simulink library "bcm"  (R2021b)
settings: Solver=VariableStepAuto  StartTime=0.0  StopTime=10.0  RelTol=1e-3
undefined symbols (not defined in the file or in its folder): ENUM_ANTITHEFT_ALARM, ENUM_ANTITHEFT_ARM, ENUM_ANTITHEFT_DISARM, ENUM_ANTITHEFT_WAIT, ENUM_GEARPOSNTOCAN_P, ENUM_PDKEYRAWLULOCK_INUNLOCK, ENUM_PDKEYRAWPS_INPS, ENUM_POWERSTA_ON, ENUM_POWERSTA_READY, ENUM_POWERSTA_STANDBY, ENUM_PWRSTASW_ON, ENUM_PWRSTASW_READY, ENUM_VEHICLETYPE_D21, ENUM_VEHICLETYPE_D31F25, ENUM_VEHICLETYPE_D31HAWD, ENUM_VEHICLETYPE_D31HRWD, ENUM_VEHICLETYPE_D31L24, FALSE, KBCM_ACCSwcPrsTmr_s, KBCM_ALMBrightnessDark_enum, KBCM_AmbBlue_enum, KBCM_AmbBreathT_ms, KBCM_AmbGreen_enum, KBCM_AmbMidPple_enum, KBCM_AmbRed_enum, KBCM_AmbTempCtrlEN_flg, KBCM_AmbTempT_s, KBCM_AmbWelModeENWait_s, KBCM_Antitheft_enum_ovrdflg, KBCM_Antitheft_enum_ovrdval, KBCM_APMDoorCtrlSta_flg_ovrdflg, KBCM_APMDoorCtrlSta_flg_ovrdval, KBCM_CmdKeepT_s, KBCM_CSWLightRstDebT_s, KBCM_CSWTurnLPRstT_s, KBCM_DelayTSW_flg, KBCM_DiagDRLOFF_flg, KBCM_DiagFLTC_mA, KBCM_DiagFMHT_s, KBCM_DiagFRTC_mA, KBCM_DiagRLTC_mA, KBCM_DiagRRTC_mA, KBCM_DrAPMRetryTimes_cnt, KBCM_DrOpenWdwOT_s, KBCM_DrOpenWdwReady_s, KBCM_ESSOffT_ms, KBCM_ESSOnT_ms, KBCM_FDCDKCReDetectT_K, KBCM_FDCDKCUSSFilterT_K, KBCM_HandleLampKeepT_s, KBCM_IVIRstHoldT_ms, KBCM_IVIRstTriggerT_ms, KBCM_ONDelayT_ms, KBCM_RAPSAbnFlashOFFT_ms, KBCM_RAPSAbnFlashONT_ms, KBCM_ReDetectT_K, KBCM_RightHandDriveEN_flg, KBCM_RLSLowSpdFilterT_s, KBCM_RmLampKeep_min, KBCM_RmLpKeyInT_s ... (+37)
libraries: simulink x389, $bdroot x11, hcu_lib x2
(part 4 of 13)

== system bcm/BCM/BCM/CenterDoorLock ==
  task_time_s : Inport
  VBCM_LockSetting_flg : Inport  Port=2
  VBCM_AntitheftSta_enum : Inport  Port=3
  VBCM_AllDoorSW_flg : Inport  Port=4  OutDataTypeStr=boolean
  VTQD_DiagHCrash_flg : Inport  Port=5
  VPMM_PwrSta_enum : Inport  Port=6
  VINP_CentralDoorLockSW_flg : Inport  Port=7
  VBCM_BCMDoorLockSta_flg : Inport  Port=8
  VBCM_ATActCtrl_enum : Inport  Port=9
  VINP_AirBagFailCmd_flg : Inport  Port=10
  VINP_VehSpeed_kph : Inport  Port=11
  VINP_funAuto_flg : Inport  Port=12
  VINP_CDLUnlockButt_flg : Inport  Port=13  OutDataTypeStr=boolean
  VINP_CDLLockButt_flg : Inport  Port=14  OutDataTypeStr=boolean
  VTQD_CrashDetd_flg : Inport  Port=15
  EEP_FuelDoorPos : Inport  Port=16
  VINP_FlashfUnlockSingle_flg : Inport  Port=17
  VINP_DrDoorSW_flg : Inport  Port=18
  VINP_PsDoorSW_flg : Inport  Port=19
  VINP_RLDoorSW_flg : Inport  Port=20
  VINP_RRDoorSW_flg : Inport  Port=21
  VINP_FLHandleClose_flg : Inport  Port=22
  VINP_FRHandleClose_flg : Inport  Port=23
  VINP_RLHandleClose_flg : Inport  Port=24
  VINP_RRHandleClose_flg : Inport  Port=25
  KBCM_CmdKeepT_s : Inport  Port=26
  KBCM_HandleLampKeepT_s : Inport  Port=27
  VTQD_ShiftGearPosn_enum : Inport  Port=28
  VBCM_AutoLockSta_flg : Inport  Port=29
  VBCM_AutoUnlockSta_flg : Inport  Port=30
  Chart : Stateflow chart  TreatAsAtomicUnit=on
      settings: PortSchema="{\"entries\":[{\"content\":{\"sides\":[{\"content\":{\"connectorIds\":[\"In24\",\"In1\",\"In2\",\"In3\",\"In25\",\"In29\",\"In26\",\"In27\",\"In28\",\"In4\",\"In5\",\"In6\",\"In7\",\"In8\",\"In9\",\"In10\",\"In11\",\"In12\",\"In13\",\"In16\",\"In19\",\"In20\",\"In22\",\"In17\",\"In18\",\"In21\",\"In23\",\"In14\",\"In15\"]},\"type\":\"ConnectorPlacement.EquallySpacedRectSide\",\"uuid\":\"d1cad239-ac39-46ec-a1da-ab943ad28110\"},{\"content\":{\"connectorIds\":[\"Out1\",\"Out2\",\"Out3\",\"Out4\",\"Out5\",\"Out6\",\"Out7\",\"Out8\",\"Out9\",\"Out10\"],\"side\":\"RIGHT\"},\"type\":\"ConnectorPlacement.EquallySpacedRectSide\",\"uuid\":\"4472ac08-1c38-4faf-8087-989b09b8fb8a\"},{\"content\":{\"connectorIds\":[],\"side\":\"TOP\"},\"type\":\"ConnectorPlacement.EquallySpacedRectSide\",\"uuid\":\"615ae9d4-02db-4768-8556-b21c6d1e705f\"}]},\"type\":\"ConnectorPlacement.EquallySpacedConnector\",\"uuid\":\"559c67f6-8021-453c-91d3-74fce83e0396\"}],\"packageUris\":[\"http://schema.mathworks.com/mf0/Connector/R2020b\"],\"version\":\"1.0\"}"
  Data Type Conversion : DataTypeConversion  OutDataTypeStr=boolean
  Data Type Conversion1 : DataTypeConversion  OutDataTypeStr=boolean
  Divide : Product  Inputs=*/
  Divide1 : Product  Inputs=*/
  Terminator : Terminator
  Unit Delay : UnitDelay  SampleTime=-1  HasFrameUpgradeWarning=on
  Unit Delay1 : UnitDelay  SampleTime=-1  HasFrameUpgradeWarning=on
  VBCM_FrChargingDoorCtrl_enum : Outport
  VBCM_RrChargingDoorCtrl_enum : Outport  Port=2
  VBCM_CrashDetd_flg : Outport  Port=3
  VBCM_CTDCtrl_enum : Outport  Port=4
  DoorLockIND : Outport  Port=5
  VBCM_fVIGHandle_flg : Outport  Port=6
  VBCM_CTDLockSW_flg : Outport  Port=7
  VBCM_FuelDoorPos_flg : Outport  Port=8
  VBCM_DiagHCrash_flg : Outport  Port=9
  VBCM_fUnlockSingle_flg : Outport  Port=10
  VBCM_FDLHandleLampCmd_flg : Outport  Port=11
  VBCM_FDRHandleLampCmd_flg : Outport  Port=12
  VBCM_FDHandleCmd_enum : Outport  Port=13
  wires:
  VBCM_AntitheftSta_enum/1 -> Chart/1(AntitheftSta)
  VINP_CDLUnlockButt_flg/1 -> Chart/9(CDL_Unlock_Butt)
  Chart/5(fVIGHandle) -> VBCM_fVIGHandle_flg/1  "VBCM_fVIGHandle_flg"
  VINP_funAuto_flg/1 -> Terminator/1
  VINP_VehSpeed_kph/1 -> Chart/8(VehSpeed)
  VINP_AirBagFailCmd_flg/1 -> Chart/7(AirBagFailCmd)
  VBCM_ATActCtrl_enum/1 -> Chart/6(ATLockCtrl)
  Chart/4(DoorLockIND) -> DoorLockIND/1  "VBCM_DoorLockIND_flg"
  VBCM_AllDoorSW_flg/1 -> Chart/2(AllDoorSW)
  Chart/1(FrChargingDoorCtrl) -> VBCM_FrChargingDoorCtrl_enum/1  "VBCM_FrChargingDoorCtrl_enum"
  Chart/2(RrChargingDoorCtrl) -> VBCM_RrChargingDoorCtrl_enum/1  "VBCM_RrChargingDoorCtrl_enum"
  VBCM_BCMDoorLockSta_flg/1 -> Chart/5(BCM_DoorLock_Sta)
  VBCM_LockSetting_flg/1 -> Chart/24(LockSetting)  "VINP_SetUnlockSingle_flg"
  Chart/3(CTDCtrl) -> VBCM_CTDCtrl_enum/1  "VBCM_CTDCtrl_enum"
  VINP_CDLLockButt_flg/1 -> Chart/10(CDL_Lock_Butt)
  [CTDLockSW] -> VBCM_CTDLockSW_flg/1  "VBCM_CTDLockSW_flg"
  VPMM_PwrSta_enum/1 -> [VPMM_PwrSta_enum]  "VPMM_PwrSta_enum"
  [VPMM_PwrSta_enum] -> Chart/3(PwrSta), Unit Delay/1
  VTQD_CrashDetd_flg/1 -> [VBCM_CrashDetd_flg]
  VINP_CentralDoorLockSW_flg/1 -> [CTDLockSW]  "VINP_CentralDoorLockSwSG09_flg"
  [CTDLockSW] -> Chart/4(CentralDoorLockSW)
  Data Type Conversion/1 -> VBCM_DiagHCrash_flg/1  "VBCM_DiagHCrash_flg"
  Data Type Conversion1/1 -> VBCM_CrashDetd_flg/1  "VBCM_CrashDetd_flg"
  VTQD_DiagHCrash_flg/1 -> Data Type Conversion/1
  [VBCM_CrashDetd_flg] -> Data Type Conversion1/1
  EEP_FuelDoorPos/1 -> Chart/12(EEP_FuelDoorPos)
  Chart/6(FuelDoorPos) -> VBCM_FuelDoorPos_flg/1  "VBCM_FuelDoorPos_flg"
  Chart/7(fUnlockSingle) -> VBCM_fUnlockSingle_flg/1  "VBCM_fUnlockSingle_flg"
  VINP_FlashfUnlockSingle_flg/1 -> Chart/13(VINP_FlashfUnlockSingle_flg)
  Chart/8(VBCM_FDLHandleLampCmd_flg) -> VBCM_FDLHandleLampCmd_flg/1
  Chart/9(VBCM_FDRHandleLampCmd_flg) -> VBCM_FDRHandleLampCmd_flg/1
  VINP_DrDoorSW_flg/1 -> Chart/16(VINP_DrDoorSW_flg)
  VINP_PsDoorSW_flg/1 -> Chart/19(VINP_PsDoorSW_flg)
  VINP_RLDoorSW_flg/1 -> Chart/20(VINP_RLDoorSW_flg)
  VINP_RRDoorSW_flg/1 -> Chart/22(VINP_RRDoorSW_flg)
  VINP_FLHandleClose_flg/1 -> Chart/17(VINP_FLHandleClose_flg)
  VINP_FRHandleClose_flg/1 -> Chart/18(VINP_FRHandleClose_flg)
  VINP_RLHandleClose_flg/1 -> Chart/21(VINP_RLHandleClose_flg)
  VINP_RRHandleClose_flg/1 -> Chart/23(VINP_RRHandleClose_flg)
  [task_time_s] -> Divide/2
  KBCM_HandleLampKeepT_s/1 -> Divide1/1
  [task_time_s] -> Divide1/2
  KBCM_CmdKeepT_s/1 -> Divide/1
  Divide/1 -> Chart/14(KBCM_CmdKeepT_s)
  Divide1/1 -> Chart/15(KBCM_HandleLampKeepT_s)
  Chart/10(VBCM_FDHandleCmd_enum) -> VBCM_FDHandleCmd_enum/1
  task_time_s/1 -> [task_time_s]
  Unit Delay/1 -> Chart/25(PwrStaBuf)
  VTQD_ShiftGearPosn_enum/1 -> Unit Delay1/1, Chart/29(VTQD_ShiftGearPosn_enum)
  Unit Delay1/1 -> Chart/26(ShiftGearPosnBuf)
  VBCM_AutoUnlockSta_flg/1 -> Chart/28(VBCM_AutoUnlockSta_flg)
  VBCM_AutoLockSta_flg/1 -> Chart/27(VBCM_AutoLockSta_flg)
  [VBCM_CrashDetd_flg] -> Chart/11(CrashDetd)

== system bcm/BCM/BCM/DID Judgement ==
  VINP_DiagFMHT_s : Inport
  VINP_DiagFLTC_mA : Inport  Port=2
  VINP_DiagFRTC_mA : Inport  Port=3
  VINP_DiagRLTC_mA : Inport  Port=4
  VINP_DiagRRTC_mA : Inport  Port=5
  VINP_DiagDRLOFF_flg : Inport  Port=6
  VINP_VehicleType_enum : Inport  Port=7
  Add1 : Sum
  Constant{,6,8,10,12,14} (6 alike) : Constant  Value=ENUM_VEHICLETYPE_D31L24
  Constant1 : Constant  Value=ENUM_VEHICLETYPE_D31HRWD
  Constant16 : Constant  Value=ENUM_VEHICLETYPE_D31F25
  Constant18 : Constant  Value=KBCM_DiagDRLOFF_flg
  Constant4 : Constant  Value=KBCM_TurnLPErrEN_flg
  Constant44 : Constant  Value=KBCM_DiagFMHT_s
  Constant45 : Constant  Value=10
  Constant46 : Constant  Value=KBCM_DiagFLTC_mA
  Constant47 : Constant  Value=KBCM_DiagFRTC_mA
  Constant48 : Constant  Value=KBCM_DiagRLTC_mA
  Constant49 : Constant  Value=KBCM_DiagRRTC_mA
  Constant7 : Constant  Value=ENUM_VEHICLETYPE_D31HAWD
  Equal{,2..9} (9 alike) : RelationalOperator  Operator===  OutDataTypeStr=boolean  RndMeth=Simplest
  Gain{,2..4} (4 alike) : Gain  Gain=10
  Gain1 : Gain  Gain=5
  Logical Operator : Logic  Operator=OR  Inputs=4  AllPortsSameDT=off  OutDataTypeStr=boolean
  Switch{,2..6} (6 alike) : Switch  Criteria=u2 > Threshold
  VBCM_DiagFMHT_s : Outport
  VBCM_DiagFLTC_mA : Outport  Port=2
  VBCM_DiagFRTC_mA : Outport  Port=3
  VBCM_DiagRLTC_mA : Outport  Port=4
  VBCM_DiagRRTC_mA : Outport  Port=5
  VBCM_DiagDRLOFF_flg : Outport  Port=6
  VBCM_TurnLPErrEN_flg : Outport  Port=7
  wires:
  Constant47/1 -> Gain2/1
  Gain1/1 -> Add1/1
  Constant45/1 -> Add1/2
  Constant49/1 -> Gain4/1
  Constant44/1 -> Gain1/1
  Constant48/1 -> Gain3/1
  Constant46/1 -> Gain/1
  [VINP_DiagFMHT_s] -> Switch/1
  Equal/1 -> Switch/2
  Add1/1 -> Switch/3
  Switch/1 -> VBCM_DiagFMHT_s/1  "VBCM_DiagFMHT_s"
  Switch6/1 -> VBCM_DiagFLTC_mA/1  "VBCM_DiagFLTC_mA"
  [VINP_DiagFLTC_mA] -> Switch6/1
  Switch2/1 -> VBCM_DiagFRTC_mA/1  "VBCM_DiagFRTC_mA"
  Gain2/1 -> Switch2/3
  [VINP_DiagFRTC_mA] -> Switch2/1
  Gain3/1 -> Switch3/3
  [VINP_DiagRLTC_mA] -> Switch3/1
  Switch3/1 -> VBCM_DiagRLTC_mA/1  "VBCM_DiagRLTC_mA"
  Gain4/1 -> Switch4/3
  [VINP_DiagRRTC_mA] -> Switch4/1
  Switch4/1 -> VBCM_DiagRRTC_mA/1  "VBCM_DiagRRTC_mA"
  Logical Operator/1 -> Switch5/2
  [VINP_DiagDRLOFF_flg] -> Switch5/1
  Switch5/1 -> VBCM_DiagDRLOFF_flg/1  "VBCM_DiagDRLOFF_flg"
  Constant18/1 -> Switch5/3
  VINP_DiagFMHT_s/1 -> [VINP_DiagFMHT_s]
  VINP_DiagFLTC_mA/1 -> [VINP_DiagFLTC_mA]
  VINP_DiagFRTC_mA/1 -> [VINP_DiagFRTC_mA]
  VINP_DiagRLTC_mA/1 -> [VINP_DiagRLTC_mA]
  VINP_DiagRRTC_mA/1 -> [VINP_DiagRRTC_mA]
  VINP_DiagDRLOFF_flg/1 -> [VINP_DiagDRLOFF_flg]
  Constant/1 -> Equal/2
  Constant6/1 -> Equal7/2
  Equal2/1 -> Switch2/2
  Constant8/1 -> Equal2/2
  Equal4/1 -> Switch3/2
  Constant12/1 -> Equal4/2
  Equal3/1 -> Switch4/2
  Constant10/1 -> Equal3/2
  Equal5/1 -> Logical Operator/1
  Constant14/1 -> Equal5/2
  Equal6/1 -> Logical Operator/2
  Constant16/1 -> Equal6/2
  VINP_VehicleType_enum/1 -> [VINP_VehicleType_enum]
  [VINP_VehicleType_enum] -> Equal/1
  [VINP_VehicleType_enum] -> Equal2/1
  [VINP_VehicleType_enum] -> Equal4/1
  [VINP_VehicleType_enum] -> Equal3/1
  [VINP_VehicleType_enum] -> Equal5/1
  [VINP_VehicleType_enum] -> Equal6/1
  [VINP_VehicleType_enum] -> Equal8/1
  Constant1/1 -> Equal8/2
  Constant7/1 -> Equal9/2
  [VINP_VehicleType_enum] -> Equal9/1
  Equal9/1 -> Logical Operator/4
  Equal8/1 -> Logical Operator/3
  Equal7/1 -> Switch6/2
  [VINP_VehicleType_enum] -> Equal7/1
  Gain/1 -> Switch6/3
  Constant4/1 -> VBCM_TurnLPErrEN_flg/1

== system bcm/BCM/BCM/Dimmer ==
  VINP_MFRDNBrightReq_pct : Inport
  VINP_IVIStatus_flg : Inport  Port=2
  VINP_IVINightModeSta_flg : Inport  Port=3
  VBCM_PosLamp_flag : Inport  Port=4
  VINP_CANMsgValidIVI2_flg : Inport  Port=5
  EEP_MFRDNBrightReq : Inport  Port=6
  BCMInitial : Inport  Port=7
  Chart : Stateflow chart  TreatAsAtomicUnit=on
      settings: PortSchema="{\"entries\":[{\"content\":{\"sides\":[{\"content\":{\"connectorIds\":[\"In4\",\"In1\",\"In2\",\"In3\"]},\"type\":\"ConnectorPlacement.EquallySpacedRectSide\",\"uuid\":\"076f305a-8f7e-4e65-8c9e-aa6699a69b21\"},{\"content\":{\"connectorIds\":[\"Out1\",\"Out2\"],\"side\":\"RIGHT\"},\"type\":\"ConnectorPlacement.EquallySpacedRectSide\",\"uuid\":\"bf947e95-3d60-4849-99c4-9fb941c8d282\"},{\"content\":{\"side\":\"TOP\"},\"type\":\"ConnectorPlacement.EquallySpacedRectSide\",\"uuid\":\"13c4efb7-da15-49ea-8253-a9d27aa3456c\"}]},\"type\":\"ConnectorPlacement.EquallySpacedConnector\",\"uuid\":\"7282b60f-551e-46a0-a3a5-beda89adbd0d\"}],\"packageUris\":[\"http://schema.mathworks.com/mf0/Connector/R2020b\"],\"version\":\"1.0\"}"
  Data Type Conversion1 : DataTypeConversion
  Switch1 : Switch  Criteria=u2 > Threshold
  Switch2 : Switch  Criteria=u2 > Threshold
  Switch3 : Switch  Criteria=u2 > Threshold
  Unit Delay : UnitDelay  SampleTime=-1  HasFrameUpgradeWarning=on
  Unit Delay1 : UnitDelay  SampleTime=-1  HasFrameUpgradeWarning=on
  VBCM_Dimmer_pct : Outport
  VBCM_DimmerEN_flg : Outport  Port=2
  VBCM_MFRDNBrightReq_pct : Outport  Port=3
  wires:
  VBCM_PosLamp_flag/1 -> Chart/3(PLamp)
  Chart/1(Dimmer) -> VBCM_Dimmer_pct/1  "VBCM_Dimmer_pct"
  VINP_IVIStatus_flg/1 -> Chart/1(IVI_Status)
  Chart/2(DimmerEN) -> VBCM_DimmerEN_flg/1  "VBCM_DimmerEN_flg"
  VINP_IVINightModeSta_flg/1 -> Switch1/1  "VINP_IVINightModeSta_flg"
  VINP_CANMsgValidIVI2_flg/1 -> Switch2/2, Switch1/2
  Switch1/1 -> Unit Delay1/1, Chart/2(IVI_Night_Mode_Sta)
  Unit Delay1/1 -> Switch1/3
  BCMInitial/1 -> Switch3/2
  EEP_MFRDNBrightReq/1 -> Switch3/3
  Switch3/1 -> Data Type Conversion1/1, Unit Delay/1
  Switch2/1 -> Switch3/1
  Unit Delay/1 -> Switch2/3
  VINP_MFRDNBrightReq_pct/1 -> Switch2/1
  Data Type Conversion1/1 -> VBCM_MFRDNBrightReq_pct/1, Chart/4(MFRD_N_Bright_Req)  "VBCM_MFRDNBrightReq_pct"

== system bcm/BCM/BCM/ExteriorLight ==
  task_time_s : Inport
  VPMM_PwrSta_enum : Inport  Port=2
  VINP_HeadLampSW_enum : Inport  Port=3
  VINP_RFogLampSW_flg : Inport  Port=4
  VINP_BrakeSWGPIO_flg : Inport  Port=5
  VINP_CSWDimSw_flg : Inport  Port=6
  VINP_CSWPassSWSta_flg : Inport  Port=7
  VTQD_ShiftGearPosn_enum : Inport  Port=8
  VBCM_OutMode_enum : Inport  Port=9
  VBCM_ATCtrl_enum : Inport  Port=10
  VINP_RLSLampSta_flg : Inport  Port=11
  VINP_ActBrkLampSta_flg : Inport  Port=12
  VINP_SRRODAWarnR_enum : Inport  Port=13
  VINP_SRRODAWarnL_enum : Inport  Port=14
  VINP_SRRBSDWarnR_enum : Inport  Port=15
  VINP_SRRBSDWarnL_enum : Inport  Port=16
  VINP_ForceLowBeam_enum : Inport  Port=17
  VINP_CANMsgValidIVI2_flg : Inport  Port=18
  VTQD_ReBrakeLPReq_flg : Inport  Port=19
  VINP_METERKPHCalcu_kph : Inport  Port=20
  VINP_DiagDRLOFF_flg : Inport  Port=21
  VINP_DiagFMHT_s : Inport  Port=22
  FDC_BCM_FollowMeENFun_Sta : Inport  Port=23
  VBCM_HLBeamENPwrSta_enum : Inport  Port=24
  VBCM_showupEN_flg : Inport  Port=25
  Chart : Stateflow chart  TreatAsAtomicUnit=on
      settings: PortSchema="{\"entries\":[{\"content\":{\"sides\":[{\"content\":{\"connectorIds\":[\"In1\",\"In2\",\"In3\",\"In4\",\"In5\",\"In6\",\"In7\",\"In8\",\"In9\",\"In10\",\"In11\",\"In12\",\"In13\",\"In14\",\"In15\",\"In16\",\"In17\",\"In18\",\"In21\",\"In19\",\"In22\",\"In20\",\"In25\",\"In23\",\"In24\"]},\"type\":\"ConnectorPlacement.EquallySpacedRectSide\",\"uuid\":\"34a74b70-26ca-4365-9514-cef344c89284\"},{\"content\":{\"connectorIds\":[\"Out1\",\"Out2\",\"Out3\",\"Out4\",\"Out5\",\"Out6\",\"Out7\",\"Out8\",\"Out9\",\"Out10\",\"Out11\",\"Out12\",\"Out13\"],\"side\":\"RIGHT\"},\"type\":\"ConnectorPlacement.EquallySpacedRectSide\",\"uuid\":\"35b33564-17af-4a68-ba31-40ca81daf0a6\"},{\"content\":{\"connectorIds\":[],\"side\":\"TOP\"},\"type\":\"ConnectorPlacement.EquallySpacedRectSide\",\"uuid\":\"ba3f7f15-bc53-4e23-8d24-280f07cf706f\"}]},\"type\":\"ConnectorPlacement.EquallySpacedConnector\",\"uuid\":\"116adca9-6a34-4fe6-9115-066bd056288e\"}],\"packageUris\":[\"http://schema.mathworks.com/mf0/Connector/R2020b\"],\"version\":\"1.0\"}"
  Constant3 : Constant  Value=KBCM_ONDelayT_ms
  Divide : Product  Inputs=*/
  HeadLampErrorHanding : Subsystem
  Switch1 : Switch  Criteria=u2 > Threshold
  Unit Delay : UnitDelay  SampleTime=-1  HasFrameUpgradeWarning=on
  Unit Delay1 : UnitDelay  SampleTime=-1  HasFrameUpgradeWarning=on
  VBCM_PosLamp_flg : Outport
  VBCM_LBeam_flg : Outport  Port=2
  VBCM_HBeam_flg : Outport  Port=3
  VBCM_RrFogLamp_flg : Outport  Port=4
  VBCM_BrakeLamp_flg : Outport  Port=5
  VBCM_ReverseLamp_flg : Outport  Port=6
  VBCM_LDRL_flg : Outport  Port=7
  VBCM_RDRL_flg : Outport  Port=8
  VBCM_LBSD_flg : Outport  Port=9
  VBCM_RBSD_flg : Outport  Port=10
  VBCM_FollowMe_flg : Outport  Port=11
  VBCM_showup_flg : Outport  Port=12
  VBCM_HBeamADB_flg : Outport  Port=13
  wires:
  Chart/11(VBCM_showup_flg) -> VBCM_showup_flg/1  "VBCM_showup_flg"
  VTQD_ReBrakeLPReq_flg/1 -> Chart/18(VTQD_ReBrakeLPReq_flg)
  VINP_DiagDRLOFF_flg/1 -> Chart/19(VBCM_DiagDRLOFF_flg)
  Unit Delay1/1 -> Switch1/3
  VINP_CANMsgValidIVI2_flg/1 -> HeadLampErrorHanding/2(VINP_CANMsgValidIVI2_flg), Switch1/2  "VINP_CANMsgValidIVI2_flg"
  Switch1/1 -> Unit Delay1/1, Chart/4(VINP_RFogLampSW_flg)
  Chart/6(VBCM_ReverseLamp_flg) -> VBCM_ReverseLamp_flg/1  "VBCM_ReverseLamp_flg"
  VTQD_ShiftGearPosn_enum/1 -> Chart/8(VTQD_ShiftGearPosn_enum)
  VINP_CSWDimSw_flg/1 -> Chart/6(VINP_CSWDimSw_flg)
  VBCM_ATCtrl_enum/1 -> Chart/10(VBCM_ATCtrl_enum)
  Chart/9(VBCM_LBSD_flg) -> VBCM_LBSD_flg/1  "VBCM_LBSD_flg"
  VINP_RLSLampSta_flg/1 -> Chart/11(VINP_RLSLampSta_flg)
  VINP_SRRBSDWarnR_enum/1 -> Chart/15(VINP_SRRBSDWarnR_enum)
  VINP_SRRBSDWarnL_enum/1 -> Chart/16(VINP_SRRBSDWarnL_enum)
  VINP_ActBrkLampSta_flg/1 -> Chart/12(VINP_ActBrkLampSta_flg)
  VINP_SRRODAWarnL_enum/1 -> Chart/14(VINP_SRRODAWarnL_enum)
  VINP_ForceLowBeam_enum/1 -> Chart/17(VINP_ForceLowBeam_enum)
  VINP_SRRODAWarnR_enum/1 -> Chart/13(VINP_SRRODAWarnR_enum)
  Chart/10(VBCM_RBSD_flg) -> VBCM_RBSD_flg/1  "VBCM_RBSD_flg"
  VBCM_OutMode_enum/1 -> Chart/9(VBCM_OutMode_enum)
  VINP_BrakeSWGPIO_flg/1 -> Chart/5(VINP_BrakeSWGPIO_flg)
  VINP_CSWPassSWSta_flg/1 -> Chart/7(VINP_CSWPassSWSta_flg)
  Chart/3(VBCM_HBeam_flg) -> VBCM_HBeam_flg/1  "VBCM_HBeam_flg"
  Chart/4(VBCM_RrFogLamp_flg) -> VBCM_RrFogLamp_flg/1  "VBCM_RrFogLamp_flg"
  VINP_RFogLampSW_flg/1 -> Switch1/1
  Chart/5(VBCM_BrakeLamp_flg) -> VBCM_BrakeLamp_flg/1  "VBCM_BrakeLamp_flg"
  Chart/2(VBCM_LBeam_flg) -> VBCM_LBeam_flg/1  "VBCM_LBeam_flg"
  Chart/7(VBCM_LDRL_flg) -> VBCM_LDRL_flg/1  "VBCM_LDRL_flg"
  Chart/8(VBCM_RDRL_flg) -> VBCM_RDRL_flg/1  "VBCM_RDRL_flg"
  VPMM_PwrSta_enum/1 -> Unit Delay/1, Chart/1(VPMM_PwrSta_enum)
  Chart/1(VBCM_PosLamp_flg) -> VBCM_PosLamp_flg/1  "VBCM_PosLamp_flg"
  VINP_METERKPHCalcu_kph/1 -> Chart/21(VINP_METERKPHCalcu_kph)
  Constant3/1 -> Chart/22(KBCM_ONDelayT_ms)
  VINP_HeadLampSW_enum/1 -> HeadLampErrorHanding/1(VINP_HeadLampSW_enum)
  HeadLampErrorHanding/1(VBCM_HeadLampSW_enum) -> Chart/3(VINP_HeadLampSW_enum)
  Chart/12(VBCM_FollowMe_flg) -> VBCM_FollowMe_flg/1  "VBCM_FollowMe_flg"
  [task_time_s] -> Divide/2
  Divide/1 -> Chart/20(VBCM_DiagFMHT_s)
  task_time_s/1 -> [task_time_s]
  VINP_DiagFMHT_s/1 -> Divide/1
  Chart/13(VBCM_HBeamADB_flg) -> VBCM_HBeamADB_flg/1  "VBCM_HBeamADB_flg"
  FDC_BCM_FollowMeENFun_Sta/1 -> Chart/25(FDC_BCM_FollowMeENFun_Sta)
  Unit Delay/1 -> Chart/2(VBCM_PwrStaBuf_enum)
  VBCM_showupEN_flg/1 -> Chart/24(VBCM_showupEN_flg)
  VBCM_HLBeamENPwrSta_enum/1 -> Chart/23(VBCM_HLBeamENPwrSta_enum)

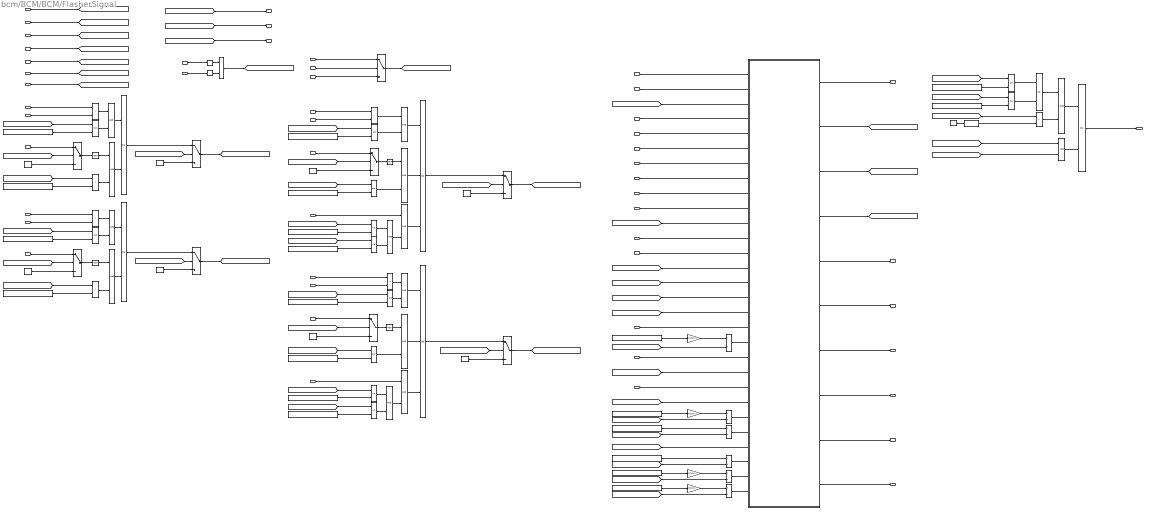
== system bcm/BCM/BCM/FlasherSignal ==
  VBCM_ATCtrl_enum : Inport
  VBCM_ATAlarm_flg : Inport  Port=2
  VPMM_PwrSta_enum : Inport  Port=3
  VINP_HazardSW_flg : Inport  Port=4
  VINP_CSWTurnSWSta_enum : Inport  Port=5
  VINP_RLTurnLampC_mA : Inport  Port=6
  VINP_RRTurnLampC_mA : Inport  Port=7
  VINP_FLTurnLampC_mA : Inport  Port=8
  VINP_FRTurnLampC_mA : Inport  Port=9
  VINP_PTGRDILsta_enum : Inport  Port=10
  VINP_ESSActive_flg : Inport  Port=11
  VINP_LeftTurnReq_flg : Inport  Port=12
  VINP_RightTurnReq_flg : Inport  Port=13
  VINP_SPTGDet_flg : Inport  Port=14
  HazardWarningReq : Inport  Port=15
  VBCM_DiagFLTC_mA : Inport  Port=16
  VBCM_DiagFRTC_mA : Inport  Port=17
  VBCM_DiagRLTC_mA : Inport  Port=18
  VBCM_DiagRRTC_mA : Inport  Port=19
  VDDM_HVRlyOpCFS_flg : Inport  Port=20
  VDDM_MCUActCFS_flg : Inport  Port=21
  task_time_s : Inport  Port=22
  VTPM_TPMSTLCmd_flg : Inport  Port=23
  VINP_CANMsgValidZONEFR1_flg : Inport  Port=24
  VINP_CANMsgValidZONEDR1_flg : Inport  Port=25
  VINP_FLTurnLPErr_flg : Inport  Port=26
  VINP_FRTurnLPErr_flg : Inport  Port=27
  VINP_RLTurnLPErr_flg : Inport  Port=28
  VINP_RRTurnLPErr_flg : Inport  Port=29
  VINP_HRLTurnLPNormalSta_flg : Inport  Port=30
  VINP_HRRTurnLPHNormalSta_flg : Inport  Port=31
  VINP_CANMsgValidZONER1_flg : Inport  Port=32
  VINP_ZRPTGRDILCmd_enum : Inport  Port=33
  VINP_RAPSBCMLamp_enum : Inport  Port=34
  VINP_APSStaSystem_enum : Inport  Port=35
  VDKC_PDKeyAreaRAPSSta_enum : Inport  Port=36
  VINP_RAPSErrWarn_enum : Inport  Port=37
  VBCM_TurnLPErrEN_flg : Inport  Port=38
  VINP_VehicleType_enum : Inport  Port=39
  VBCM_UnlockWelcomeEN_flg : Inport  Port=40
  AND : Logic  AllPortsSameDT=off  OutDataTypeStr=boolean
  Chart : Stateflow chart  TreatAsAtomicUnit=on
      settings: PortSchema="{\"entries\":[{\"content\":{\"sides\":[{\"content\":{\"connectorIds\":[\"In1\",\"In2\",\"In3\",\"In4\",\"In5\",\"In7\",\"In8\",\"In9\",\"In10\",\"In11\",\"In6\",\"In12\",\"In13\",\"In23\",\"In22\",\"In17\",\"In18\",\"In16\",\"In14\",\"In27\",\"In28\",\"In29\",\"In24\",\"In15\",\"In19\",\"In21\",\"In20\",\"In26\",\"In25\"]},\"type\":\"ConnectorPlacement.EquallySpacedRectSide\",\"uuid\":\"fb222101-3ebe-4085-bdf3-20ef70df8d28\"},{\"content\":{\"connectorIds\":[\"Out1\",\"Out2\",\"Out3\",\"Out4\",\"Out5\",\"Out6\",\"Out7\",\"Out8\",\"Out9\",\"Out10\"],\"side\":\"RIGHT\"},\"type\":\"ConnectorPlacement.EquallySpacedRectSide\",\"uuid\":\"1d165777-adb5-42aa-9b79-2429bdff6c1c\"},{\"content\":{\"connectorIds\":[],\"side\":\"TOP\"},\"type\":\"ConnectorPlacement.EquallySpacedRectSide\",\"uuid\":\"46eb436b-9b3b-4f68-9e11-94686797b079\"}]},\"type\":\"ConnectorPlacement.EquallySpacedConnector\",\"uuid\":\"ccb97afc-e3e1-4b58-940d-fbdbd7472620\"}],\"packageUris\":[\"http://schema.mathworks.com/mf0/Connector/R2020b\"],\"version\":\"1.0\"}"
  Compare To Constant : simulink/Logic and Bit Operations/Compare To Constant  relop=~=  const=1  OutDataTypeStr=boolean
  Compare To Constant1 : simulink/Logic and Bit Operations/Compare To Constant  relop===  const=4  OutDataTypeStr=boolean
  Constant : Constant  Value=KBCM_ESSOnT_ms
  Constant1 : Constant  Value=KBCM_ESSOffT_ms
  Constant{8,10..12,14..15,25..26} (8 alike) : Constant  Value=TRUE
  Constant{7,9,13,16,19,23,27,29} (8 alike) : Constant  Value=ENUM_VEHICLETYPE_D31L24
  Constant2 : Constant  Value=3
  Constant20 : Constant  Value=KBCM_RAPSAbnFlashOFFT_ms
  Constant21 : Constant  Value=KBCM_RAPSAbnFlashONT_ms
  Constant{22,24,28,30} (4 alike) : Constant  Value=ENUM_VEHICLETYPE_D21
  Constant3 : Constant  Value=ENUM_POWERSTA_ON
  Constant4 : Constant  Value=ENUM_POWERSTA_READY
  Constant5 : Constant  Value=KBCM_WelcomeT_s
  Constant6 : Constant  Value=KBCM_WelLockT_s
  Data Type Conversion : DataTypeConversion  OutDataTypeStr=uint8
  Divide{,1..5} (6 alike) : Product  Inputs=*/
  Equal : RelationalOperator  Operator===  OutDataTypeStr=boolean  RndMeth=Simplest
  Equal1 : RelationalOperator  Operator===  OutDataTypeStr=boolean  RndMeth=Simplest
  Gain{,1..3} (4 alike) : Gain  Gain=XX2KXX
  Less Than{,1..2,5,7,14} (6 alike) : RelationalOperator  Operator=>  OutDataTypeStr=boolean  RndMeth=Simplest
  Less Than{10..13} (4 alike) : RelationalOperator  Operator=~=  OutDataTypeStr=boolean  RndMeth=Simplest
  Less Than{4,6,8..9,15..16} (6 alike) : RelationalOperator  Operator===  OutDataTypeStr=boolean  RndMeth=Simplest
  Logical Operator : Logic  AllPortsSameDT=off  OutDataTypeStr=boolean
  Logical Operator1 : Logic  Operator=OR  AllPortsSameDT=off  OutDataTypeStr=boolean
  Logical Operator2 : Logic  AllPortsSameDT=off  OutDataTypeStr=boolean
  Logical Operator3 : Logic  Operator=OR  AllPortsSameDT=off  OutDataTypeStr=boolean
  NOT{,1..2,4} (4 alike) : Logic  Operator=NOT  AllPortsSameDT=off  OutDataTypeStr=boolean
  OR : Logic  Operator=OR  AllPortsSameDT=off  OutDataTypeStr=boolean
  OR1 : Logic  Operator=OR  AllPortsSameDT=off  OutDataTypeStr=boolean
  OR{4..13,15..16} (12 alike) : Logic  AllPortsSameDT=off  OutDataTypeStr=boolean
  OR14 : Logic  Operator=OR  Inputs=3  AllPortsSameDT=off  OutDataTypeStr=boolean
  OR2 : Logic  Operator=OR  Inputs=3  AllPortsSameDT=off  OutDataTypeStr=boolean
  Relational Operator : RelationalOperator  Operator=<  OutDataTypeStr=boolean  RndMeth=Simplest
  Switch{,1..5,9..10} (8 alike) : Switch  Criteria=u2 ~= 0
  Switch8 : Switch  Criteria=u2 > Threshold
  VBCM_HazardSW_flg : Outport
  VBCM_LTurnLP_flg : Outport  Port=2
  VBCM_RTurnLP_flg : Outport  Port=3
  VBCM_OutMode_enum : Outport  Port=4
  VBCM_BCMBuzzerReq_flg : Outport  Port=5
  VBCM_DiagFLTS_flg : Outport  Port=6
  VBCM_DiagFRTS_flg : Outport  Port=7
  VBCM_DiagRLTS_flg : Outport  Port=8
  VBCM_DiagRRTS_flg : Outport  Port=9
  VBCM_HazardIND_flg : Outport  Port=10
  VBCM_WelcomeLight_enum : Outport  Port=11
  wires:
  Chart/1(HazardSW) -> VBCM_HazardSW_flg/1  "VBCM_HazardSW_flg"
  VBCM_ATCtrl_enum/1 -> Chart/1(ATCtrl)
  VINP_HazardSW_flg/1 -> Chart/4(HazardSWSta)
  VBCM_ATAlarm_flg/1 -> Chart/2(ATAlarm)
  VINP_CSWTurnSWSta_enum/1 -> Chart/5(CSW_TurnSw_Sta)
  VINP_ESSActive_flg/1 -> Chart/7(ESS_Active)
  VINP_LeftTurnReq_flg/1 -> Chart/8(LeftTurnLightReq)
  VINP_RightTurnReq_flg/1 -> Chart/9(RightTurnLightReq)
  VINP_PTGRDILsta_enum/1 -> Switch8/3
  HazardWarningReq/1 -> Chart/11(HazardWarningReq)
  VINP_SPTGDet_flg/1 -> Chart/10(SPTGDet)
  Chart/9(BCMBuzzerReq) -> VBCM_BCMBuzzerReq_flg/1  "VBCM_BCMBuzzerReq_flg"
  VDDM_HVRlyOpCFS_flg/1 -> Chart/12(VDDM_HVRlyOpCFS_flg)
  VDDM_MCUActCFS_flg/1 -> Chart/13(VDDM_MCUActCFS_flg)
  Chart/6(DiagFRTS) -> VBCM_DiagFRTS_flg/1  "VBCM_DiagFRTS_flg"
  Chart/7(DiagRLTS) -> VBCM_DiagRLTS_flg/1  "VBCM_DiagRLTS_flg"
  Chart/5(DiagFLTS) -> VBCM_DiagFLTS_flg/1  "VBCM_DiagFLTS_flg"
  Chart/8(DiagRRTS) -> VBCM_DiagRRTS_flg/1  "VBCM_DiagRRTS_flg"
  Constant/1 -> Gain/1
  [task_time_s] -> Divide/2
  Gain/1 -> Divide/1
  Divide/1 -> Chart/14(VBCM_ESSOnT_tick)
  Divide1/1 -> Chart/15(VBCM_ESSOffT_tick)
  [task_time_s] -> Divide1/2
  Gain1/1 -> Divide1/1
  Constant1/1 -> Gain1/1
  task_time_s/1 -> [task_time_s]
  VPMM_PwrSta_enum/1 -> [VPMM_PwrSta_enum]
  [VPMM_PwrSta_enum] -> Chart/3(PwrSta)
  Chart/4(OutMode) -> [VBCM_OutMode_enum]  "VBCM_OutMode_enum"
  [VBCM_OutMode_enum] -> VBCM_OutMode_enum/1
  Chart/2(LTurnLP) -> [VBCM_LTurnLP_flg]  "VBCM_LTurnLP_flg"
  Chart/3(RTurnLP) -> [VBCM_RTurnLP_flg]  "VBCM_RTurnLP_flg"
  [VBCM_LTurnLP_flg] -> VBCM_LTurnLP_flg/1
  [VBCM_RTurnLP_flg] -> VBCM_RTurnLP_flg/1
  [VBCM_LTurnLP_flg] -> Logical Operator/1
  [VBCM_RTurnLP_flg] -> Logical Operator/2
  Constant2/1 -> Data Type Conversion/1
  Data Type Conversion/1 -> Relational Operator/2
  [VBCM_OutMode_enum] -> Relational Operator/1
  [VPMM_PwrSta_enum] -> Equal/1
  Constant3/1 -> Equal/2
  Constant4/1 -> Equal1/2
  [VPMM_PwrSta_enum] -> Equal1/1
  Equal/1 -> Logical Operator1/1
  Equal1/1 -> Logical Operator1/2
  Logical Operator1/1 -> Logical Operator2/1
  Relational Operator/1 -> Logical Operator2/2
  Logical Operator2/1 -> Logical Operator3/1
  Logical Operator/1 -> Logical Operator3/2
  Logical Operator3/1 -> VBCM_HazardIND_flg/1  "VBCM_HazardIND_flg"
  VTPM_TPMSTLCmd_flg/1 -> Chart/16(VTPM_TPMSTLCmd_flg)
  [task_time_s] -> Divide2/2
  Constant5/1 -> Divide2/1
  Divide2/1 -> Chart/19(KBCM_WelcomeT_s)
  Divide3/1 -> Chart/20(KBCM_WelLockT_s)
  Constant6/1 -> Divide3/1
  [task_time_s] -> Divide3/2
  VINP_FLTurnLampC_mA/1 -> Less Than/1
  VBCM_DiagFLTC_mA/1 -> Less Than/2
  Switch/1 -> NOT/1
  VINP_FLTurnLPErr_flg/1 -> Switch/1
  VINP_CANMsgValidZONEFR1_flg/1 -> [VINP_CANMsgValidZONEFR1_flg]
  [VINP_CANMsgValidZONEFR1_flg] -> Switch/2
  Constant8/1 -> Switch/3
  OR/1 -> Switch1/1
  Constant10/1 -> Switch1/3
  Switch1/1 -> [VBCM_FLTurnLPNormal_flg]
  Switch3/1 -> [VBCM_FRTurnLPNormal_flg]
  Constant11/1 -> Switch3/3
  [VBCM_TurnLPErrEN_flg] -> Switch3/2
  OR1/1 -> Switch3/1
  Constant12/1 -> Switch2/3
  [VINP_CANMsgValidZONEFR1_flg] -> Switch2/2
  Switch2/1 -> NOT1/1
  VINP_FRTurnLampC_mA/1 -> Less Than1/1
  VBCM_DiagFRTC_mA/1 -> Less Than1/2
  VINP_FRTurnLPErr_flg/1 -> Switch2/1
  VINP_RLTurnLPErr_flg/1 -> Switch4/1
  Switch4/1 -> NOT2/1
  [VINP_CANMsgValidZONEDR1_flg] -> Switch4/2
  Constant15/1 -> Switch4/3
  OR2/1 -> Switch5/1
  [VBCM_TurnLPErrEN_flg] -> Switch5/2
  Constant14/1 -> Switch5/3
  Switch5/1 -> [VBCM_RLTurnLPNormal_flg]
  [VBCM_FLTurnLPNormal_flg] -> Chart/23(FLTurnLPNormal)
  [VBCM_FRTurnLPNormal_flg] -> Chart/22(FRTurnLPNormal)
  VBCM_DiagRLTC_mA/1 -> Less Than2/2
  VINP_RLTurnLampC_mA/1 -> Less Than2/1
  VINP_CANMsgValidZONEDR1_flg/1 -> [VINP_CANMsgValidZONEDR1_flg]
  [VBCM_RLTurnLPNormal_flg] -> Chart/17(RLTurnLPNormal)
  [VBCM_RRTurnLPNormal_flg] -> Chart/18(RRTurnLPNormal)
  Chart/10(WelcomeLight) -> VBCM_WelcomeLight_enum/1  "VBCM_WelcomeLight_enum"
  VINP_ZRPTGRDILCmd_enum/1 -> Switch8/1
  Switch8/1 -> [VBCM_PTGRDIL_enum]
  VINP_CANMsgValidZONER1_flg/1 -> Switch8/2
  [VBCM_PTGRDIL_enum] -> Chart/6(PTG_RDIL_Sta)
  Compare To Constant/1 -> AND/1
  VDKC_PDKeyAreaRAPSSta_enum/1 -> Compare To Constant/1
  AND/1 -> [VBCM_RAPSAbnFlashReq_flg]
  Compare To Constant1/1 -> AND/2
  VINP_APSStaSystem_enum/1 -> Compare To Constant1/1
  Divide5/1 -> Chart/26(KBCM_RAPSAbnFlashONT_ms)
  Constant21/1 -> Gain3/1
  [task_time_s] -> Divide4/2
  Gain2/1 -> Divide4/1
  Constant20/1 -> Gain2/1
  [task_time_s] -> Divide5/2
  Gain3/1 -> Divide5/1
  Divide4/1 -> Chart/25(KBCM_RAPSAbnFlashOFFT_ms)
  VINP_RAPSErrWarn_enum/1 -> Chart/29(VINP_RAPSErrWarn_enum)
  VINP_RAPSBCMLamp_enum/1 -> Chart/27(RAPSBCMLampCmd)
  [VBCM_RAPSAbnFlashReq_flg] -> Chart/28(VBCM_RAPSAbnFlashReq_flg)
  VBCM_TurnLPErrEN_flg/1 -> [VBCM_TurnLPErrEN_flg]
  [VBCM_TurnLPErrEN_flg] -> Switch1/2
  VINP_VehicleType_enum/1 -> [VINP_VehicleType_enum]
  [VINP_VehicleType_enum] -> Chart/21(VINP_VehicleType_enum)
  Less Than/1 -> OR4/1
  Less Than4/1 -> OR4/2
  [VINP_VehicleType_enum] -> Less Than4/1
  Constant7/1 -> Less Than4/2
  NOT/1 -> OR5/1
  OR4/1 -> OR/1
  OR5/1 -> OR/2
  Constant9/1 -> Less Than5/2
  [VINP_VehicleType_enum] -> Less Than5/1
  Less Than5/1 -> OR5/2
  OR6/1 -> OR1/2
  NOT1/1 -> OR6/1
  Constant13/1 -> Less Than6/2
  [VINP_VehicleType_enum] -> Less Than6/1
  Less Than6/1 -> OR7/2
  OR7/1 -> OR1/1
  Less Than1/1 -> OR7/1
  Less Than7/1 -> OR6/2
  [VINP_VehicleType_enum] -> Less Than7/1
  Constant16/1 -> Less Than7/2
  Constant19/1 -> Less Than8/2
  [VINP_VehicleType_enum] -> Less Than8/1
  Less Than8/1 -> OR8/2
  OR8/1 -> OR2/1
  Less Than2/1 -> OR8/1
  Less Than9/1 -> OR9/2
  [VINP_VehicleType_enum] -> Less Than9/1
  Constant22/1 -> Less Than9/2
  OR9/1 -> OR2/2
  NOT2/1 -> OR9/1
  OR10/1 -> OR2/3
  VINP_HRLTurnLPNormalSta_flg/1 -> OR10/1
  OR11/1 -> OR10/2
  Constant23/1 -> Less Than10/2
  [VINP_VehicleType_enum] -> Less Than10/1
  [VINP_VehicleType_enum] -> Less Than11/1
  Constant24/1 -> Less Than11/2
  Less Than10/1 -> OR11/1
  Less Than11/1 -> OR11/2
  Less Than13/1 -> OR13/2
  Less Than12/1 -> OR13/1
  Constant30/1 -> Less Than13/2
  [VINP_VehicleType_enum] -> Less Than13/1
  [VINP_VehicleType_enum] -> Less Than12/1
  Constant29/1 -> Less Than12/2
  OR13/1 -> OR12/2
  OR12/1 -> OR14/3
  NOT4/1 -> OR16/1
  OR16/1 -> OR14/2
  Constant28/1 -> Less Than16/2
  [VINP_VehicleType_enum] -> Less Than16/1
  Less Than16/1 -> OR16/2
  Less Than14/1 -> OR15/1
  OR15/1 -> OR14/1
  Less Than15/1 -> OR15/2
  [VINP_VehicleType_enum] -> Less Than15/1
  Constant27/1 -> Less Than15/2
  Constant25/1 -> Switch10/3
  [VBCM_TurnLPErrEN_flg] -> Switch10/2
  OR14/1 -> Switch10/1
  Constant26/1 -> Switch9/3
  [VINP_CANMsgValidZONEDR1_flg] -> Switch9/2
  Switch9/1 -> NOT4/1
  Switch10/1 -> [VBCM_RRTurnLPNormal_flg]
  VINP_RRTurnLampC_mA/1 -> Less Than14/1
  VBCM_DiagRRTC_mA/1 -> Less Than14/2
  VINP_HRRTurnLPHNormalSta_flg/1 -> OR12/1
  VINP_RRTurnLPErr_flg/1 -> Switch9/1
  VBCM_UnlockWelcomeEN_flg/1 -> [VBCM_UnlockWelcomeEN_flg]
  [VBCM_UnlockWelcomeEN_flg] -> Chart/24(VBCM_UnlockWelcomeEN_flg)

== system bcm/BCM/BCM/HMI_Custom_Button ==
  VINP_IVIHMICustmiKEYSta_enum : Inport
  VINP_IVIHMICustmiFunSta_enum : Inport  Port=2
  VINP_FlashHMIKey1Func_enum : Inport  Port=3
  VINP_FlashHMIKey2Func_enum : Inport  Port=4
  VINP_FlashHMIKey3Func_enum : Inport  Port=5
  VINP_FlashHMIKey4Func_enum : Inport  Port=6
  VINP_FlashHMIKey5Func_enum : Inport  Port=7
  VINP_FlashHMIKey6Func_enum : Inport  Port=8
  VINP_FlashHMIKey7Func_enum : Inport  Port=9
  VINP_FlashHMIKey8Func_enum : Inport  Port=10
  Constant : Constant  Value=TRUE
  Constant1 : Constant
  Constant10 : Constant  Value=2
  Constant11 : Constant  Value=3
  Constant12 : Constant  Value=4
  Constant13 : Constant  Value=4
  Constant14 : Constant  Value=6
  Constant15 : Constant  Value=5
  Constant16 : Constant  Value=6
  Constant17 : Constant  Value=8
  Constant18 : Constant  Value=8
  Constant19 : Constant  Value=7
  Constant2 : Constant
  Constant20 : Constant  Value=2
  Constant3 : Constant  Value=3
  Constant4 : Constant  Value=5
  Constant5 : Constant  Value=7
  Data Type Conversion{,1..7} (8 alike) : DataTypeConversion  OutDataTypeStr=uint8
  Key1 : Subsystem
  Key{2..8} (7 alike) : $bdroot/BCM/BCM/HMI_Custom_Button/Key1  SystemSampleTime=-1  VariantActivationTime=update diagram  Latency=0  AutoFrameSizeCalculation=off
  Unit Delay : UnitDelay  SampleTime=-1  HasFrameUpgradeWarning=on
  Unit Delay1 : UnitDelay  SampleTime=-1  HasFrameUpgradeWarning=on
  VBCM_HMIKey1FuncSta_enum : Outport
  VBCM_HMIKey2FuncSta_enum : Outport  Port=2
  VBCM_HMIKey3FuncSta_enum : Outport  Port=3
  VBCM_HMIKey4FuncSta_enum : Outport  Port=4
  VBCM_HMIKey5FuncSta_enum : Outport  Port=5
  VBCM_HMIKey6FuncSta_enum : Outport  Port=6
  VBCM_HMIKey7FuncSta_enum : Outport  Port=7
  VBCM_HMIKey8FuncSta_enum : Outport  Port=8
  wires:
  Constant/1 -> Unit Delay/1
  Unit Delay/1 -> Unit Delay1/1
  Unit Delay1/1 -> [InitialBar]
  [InitialBar] -> Key1/6(InitialBar)
  Constant1/1 -> Key1/1(KeyNum)
  VINP_IVIHMICustmiKEYSta_enum/1 -> [VINP_IVIHMICustmiKEYSta_enum]
  VINP_IVIHMICustmiFunSta_enum/1 -> [VINP_IVIHMICustmiFunSta_enum]
  [VINP_IVIHMICustmiKEYSta_enum] -> Key1/2(IVI_HMICustmKEY_Sta)
  [VINP_IVIHMICustmiFunSta_enum] -> Key1/3(IVI_HMICustmFun_Sta)
  VINP_FlashHMIKey1Func_enum/1 -> Key1/4(KeyFuncMem)
  Constant2/1 -> Data Type Conversion/1
  Data Type Conversion/1 -> Key1/5(PreSetFunc)
  Key1/1(KeyFunc) -> VBCM_HMIKey1FuncSta_enum/1
  Constant11/1 -> Data Type Conversion1/1
  VINP_FlashHMIKey2Func_enum/1 -> Key2/4
  Constant10/1 -> Key2/1
  [InitialBar] -> Key2/6
  [VINP_IVIHMICustmiKEYSta_enum] -> Key2/2
  [VINP_IVIHMICustmiFunSta_enum] -> Key2/3
  Data Type Conversion1/1 -> Key2/5
  Key2/1 -> VBCM_HMIKey2FuncSta_enum/1
  [InitialBar] -> Key3/6
  Constant3/1 -> Key3/1
  VINP_FlashHMIKey3Func_enum/1 -> Key3/4
  Constant12/1 -> Data Type Conversion2/1
  [VINP_IVIHMICustmiKEYSta_enum] -> Key3/2
  [VINP_IVIHMICustmiFunSta_enum] -> Key3/3
  Data Type Conversion2/1 -> Key3/5
  Key3/1 -> VBCM_HMIKey3FuncSta_enum/1
  Key4/1 -> VBCM_HMIKey4FuncSta_enum/1
  [VINP_IVIHMICustmiFunSta_enum] -> Key4/3
  [VINP_IVIHMICustmiKEYSta_enum] -> Key4/2
  Constant5/1 -> Data Type Conversion3/1
  VINP_FlashHMIKey4Func_enum/1 -> Key4/4
  Constant13/1 -> Key4/1
  [InitialBar] -> Key4/6
  Data Type Conversion3/1 -> Key4/5
  Key8/1 -> VBCM_HMIKey8FuncSta_enum/1
  Key7/1 -> VBCM_HMIKey7FuncSta_enum/1
  Key6/1 -> VBCM_HMIKey6FuncSta_enum/1
  Key5/1 -> VBCM_HMIKey5FuncSta_enum/1
  [InitialBar] -> Key8/6
  Constant17/1 -> Key8/1
  VINP_FlashHMIKey8Func_enum/1 -> Key8/4
  Constant20/1 -> Data Type Conversion7/1
  Constant16/1 -> Data Type Conversion6/1
  VINP_FlashHMIKey7Func_enum/1 -> Key7/4
  Constant19/1 -> Key7/1
  [InitialBar] -> Key7/6
  [InitialBar] -> Key6/6
  Constant14/1 -> Key6/1
  VINP_FlashHMIKey6Func_enum/1 -> Key6/4
  Constant15/1 -> Data Type Conversion5/1
  Constant18/1 -> Data Type Conversion4/1
  VINP_FlashHMIKey5Func_enum/1 -> Key5/4
  Constant4/1 -> Key5/1
  [InitialBar] -> Key5/6
  [VINP_IVIHMICustmiKEYSta_enum] -> Key5/2
  [VINP_IVIHMICustmiFunSta_enum] -> Key5/3
  Data Type Conversion4/1 -> Key5/5
  [VINP_IVIHMICustmiKEYSta_enum] -> Key6/2
  [VINP_IVIHMICustmiFunSta_enum] -> Key6/3
  Data Type Conversion5/1 -> Key6/5
  [VINP_IVIHMICustmiKEYSta_enum] -> Key7/2
  [VINP_IVIHMICustmiFunSta_enum] -> Key7/3
  Data Type Conversion6/1 -> Key7/5
  [VINP_IVIHMICustmiKEYSta_enum] -> Key8/2
  [VINP_IVIHMICustmiFunSta_enum] -> Key8/3
  Data Type Conversion7/1 -> Key8/5

== system bcm/BCM/BCM/IVI Reset ==
  VINP_SWCmodeSta_flg : Inport
  KBCM_IVIRstHoldT_ms : Inport  Port=2
  KBCM_IVIRstTriggerT_ms : Inport  Port=3
  Chart : Stateflow chart  TreatAsAtomicUnit=on
      settings: PortSchema="{\"entries\":[{\"content\":{\"sides\":[{\"content\":{\"connectorIds\":[\"In3\",\"In1\",\"In2\"]},\"type\":\"ConnectorPlacement.EquallySpacedRectSide\",\"uuid\":\"527c4af8-44de-47f2-8701-d5f5b7b571d6\"},{\"content\":{\"connectorIds\":[\"Out1\"],\"side\":\"RIGHT\"},\"type\":\"ConnectorPlacement.EquallySpacedRectSide\",\"uuid\":\"5335a623-2c87-4967-8624-b1c657e6893f\"},{\"content\":{\"connectorIds\":[],\"side\":\"TOP\"},\"type\":\"ConnectorPlacement.EquallySpacedRectSide\",\"uuid\":\"ed42b152-df02-4687-bffb-78347cddc5c0\"}]},\"type\":\"ConnectorPlacement.EquallySpacedConnector\",\"uuid\":\"716ba71d-aae5-4637-96c7-fec6e8a69169\"}],\"packageUris\":[\"http://schema.mathworks.com/mf0/Connector/R2020b\"],\"version\":\"1.0\"}"
  Gain : Gain  Gain=1/10
  Gain1 : Gain  Gain=1/10
  Ground : Ground
  Terminator : Terminator
  VBCM_IVIRST_flg : Outport
  wires:
  KBCM_IVIRstHoldT_ms/1 -> Gain/1
  KBCM_IVIRstTriggerT_ms/1 -> Gain1/1
  VINP_SWCmodeSta_flg/1 -> Chart/3(VINP_SWCmodeSta_flg)
  Gain/1 -> Chart/1(KBCM_IVIRstHoldT_ms)
  Gain1/1 -> Chart/2(KBCM_IVIRstTriggerT_ms)
  Chart/1(VBCM_IVIRST_flg) -> Terminator/1
  Ground/1 -> VBCM_IVIRST_flg/1  "VBCM_IVIRST_flg"

== system bcm/BCM/BCM/PTG ==
  note: Modify Part
  task_time_s : Inport
  VINP_PDKeyAreaPTG_enum : Inport  Port=2
  VDKC_KeyAreaSPTGSta_enum : Inport  Port=3
  VINP_TailgateSW_flg : Inport  Port=4
  VAPM_PASDRMR_cm : Inport  Port=5
  VAPM_PASDRML_cm : Inport  Port=6
  VINP_PCommandToBCM_enum : Inport  Port=7
  VPMM_PwrSta_eunm : Inport  Port=8
  VTQD_ShiftGearPosn_enum : Inport  Port=9
  VBCM_SPTGENFun_flg : Inport  Port=10
  VINP_VehSpeed_kph : Inport  Port=11
  KBCM_DelayTSW_flg : Inport  Port=12
  KBCM_ReDetectT_K : Inport  Port=13
  KBCM_SPTGDetectT_sec : Inport  Port=14
  KBCM_SPTGLeave_flg : Inport  Port=15
  KBCM_SPTGWaitDKC_sec : Inport  Port=16
  VINP_VehicleType_enum : Inport  Port=17
  AND : Logic  AllPortsSameDT=off  OutDataTypeStr=boolean
  AND1 : Logic  AllPortsSameDT=off  OutDataTypeStr=boolean
  Add1 : Sum
  Chart : Stateflow chart  TreatAsAtomicUnit=on
      settings: PortSchema="{\"entries\":[{\"content\":{\"sides\":[{\"content\":{\"connectorIds\":[\"In1\",\"In13\",\"In14\",\"In15\",\"In16\",\"In3\",\"In2\",\"In7\",\"In5\",\"In4\",\"In6\",\"In8\",\"In9\",\"In10\",\"In11\",\"In12\",\"In17\"]},\"type\":\"ConnectorPlacement.EquallySpacedRectSide\",\"uuid\":\"2c0d242d-6a76-4137-8e1d-4d6809bc83cf\"},{\"content\":{\"connectorIds\":[\"Out2\",\"Out1\"],\"side\":\"RIGHT\"},\"type\":\"ConnectorPlacement.EquallySpacedRectSide\",\"uuid\":\"af4f90f4-f68e-4fa9-bb59-784446720a84\"},{\"content\":{\"connectorIds\":[],\"side\":\"TOP\"},\"type\":\"ConnectorPlacement.EquallySpacedRectSide\",\"uuid\":\"f397bac8-7d09-437c-83a0-3821a6ac718f\"}]},\"type\":\"ConnectorPlacement.EquallySpacedConnector\",\"uuid\":\"a750c59f-e2db-4dfa-b2ae-496db5c88784\"}],\"packageUris\":[\"http://schema.mathworks.com/mf0/Connector/R2020b\"],\"version\":\"1.0\"}"
  Compare To Constant{,1..2,4..5} (5 alike) : simulink/Logic and Bit Operations/Compare To Constant  relop===  const=1  OutDataTypeStr=boolean
  Compare To Constant3 : simulink/Logic and Bit Operations/Compare To Constant  relop=<  const=KBCM_SPTGLowerBound_cm  OutDataTypeStr=boolean
  Compare To Constant6 : simulink/Logic and Bit Operations/Compare To Constant  relop=<  const=KBCM_SPTGLowerBound_cm  OutDataTypeStr=boolean
  Constant : Constant  Value=KBCM_SPTGDetectWaitT_s
  Constant1 : Constant  Value=95
  Constant10 : Constant  Value=0
  Constant11 : Constant  Value=0
  Constant12 : Constant  Value=KBCM_SPTGZoneRejectEN_flg
  Constant19 : Constant  Value=KBCM_FDCDKCUSSFilterT_K
  Constant2 : Constant  Value=ENUM_VEHICLETYPE_D31L24
  Constant3 : Constant  Value=FALSE
  Constant4 : Constant  Value=TRUE
  Constant5 : Constant  Value=KBCM_USSFilterT_K
  Constant6 : Constant  Value=70
  Constant7 : Constant  Value=KBCM_FDCDKCReDetectT_K
  Constant8 : Constant  Value=200
  Constant9 : Constant  Value=KBCM_SPTGZoneDebT_s
  Data Type Conversion{1..2,5,7} (4 alike) : DataTypeConversion  OutDataTypeStr=uint8
  Data Type Conversion3 : DataTypeConversion  OutDataTypeStr=single
  Detect Change : simulink/Logic and Bit Operations/Detect Change  vinit=0  OutDataTypeStr=boolean
  Detect Change2 : simulink/Logic and Bit Operations/Detect Change  vinit=0  OutDataTypeStr=boolean
  Divide : Product  Inputs=*/
  Equal : RelationalOperator  Operator===  OutDataTypeStr=boolean  RndMeth=Simplest
  KeyDetected : Subsystem
  Less Than1 : RelationalOperator  Operator=<  OutDataTypeStr=boolean  RndMeth=Simplest
  NOT : Logic  Operator=NOT  AllPortsSameDT=off  OutDataTypeStr=boolean
  OR : Logic  Operator=OR  AllPortsSameDT=off  OutDataTypeStr=boolean
  Saturation1 : Saturate  UpperLimit=KBCM_SPTGZoneDebT_s  LowerLimit=0
  Subsystem1 : Subsystem
  Subsystem3 : Subsystem
  Switch : Switch  Criteria=u2 > Threshold
  Switch{1..5,7..11} (10 alike) : Switch  Criteria=u2 ~= 0
  Switch6 : Switch  Criteria=u2 > Threshold
  Unit Delay2 : UnitDelay  SampleTime=-1  HasFrameUpgradeWarning=on
  Unit Delay3 : UnitDelay  SampleTime=-1  HasFrameUpgradeWarning=on
  VBCM_SPTGDet_flg : Outport
  VBCM_APSOpenPTG_flg : Outport  Port=2
  wires:
  KeyDetected/1(KeyDetected) -> Switch3/1, Chart/2(KeyDetected)  "VBCM_PASKeyDetected_flg"
  VINP_VehSpeed_kph/1 -> Chart/9(VehSpeed)
  VINP_PCommandToBCM_enum/1 -> Detect Change/1
  VTQD_ShiftGearPosn_enum/1 -> Chart/11(ShiftGearPosn)
  VINP_TailgateSW_flg/1 -> Chart/8(TailgateSW)
  Chart/1(VBCM_APSOpenPTG_flg) -> VBCM_APSOpenPTG_flg/1
  Detect Change/1 -> Chart/10(DKCKeyPress)  "DKCKeyPress"
  VPMM_PwrSta_eunm/1 -> Chart/6(PwrSta)
  Chart/2(VBCM_SPTGDet_flg) -> VBCM_SPTGDet_flg/1
  KBCM_DelayTSW_flg/1 -> Chart/1(KBCM_DelayTSW_flg)
  KBCM_SPTGDetectT_sec/1 -> Chart/14(KBCM_SPTGDetectT_sec)
  KBCM_SPTGLeave_flg/1 -> Chart/15(KBCM_SPTGLeave_flg)
  Compare To Constant/1 -> Chart/5(PDKeyAreaPTG)
  KBCM_SPTGWaitDKC_sec/1 -> Chart/16(KBCM_SPTGWaitDKC_sec)
  VBCM_SPTGENFun_flg/1 -> NOT/1
  NOT/1 -> Chart/12(IVI_PTG_USSta_SW)
  [VBCM_FDCDKCEn_flg] -> Switch1/2
  [VBCM_FDCDKCEn_flg] -> Switch2/2
  Switch4/1 -> Switch2/1, Switch1/1
  Compare To Constant1/1 -> Switch4/2
  Data Type Conversion5/1 -> Switch4/1
  Constant6/1 -> Data Type Conversion5/1
  Constant8/1 -> Data Type Conversion7/1
  Constant2/1 -> Equal/2
  Equal/1 -> Switch/2
  Constant4/1 -> Switch/3
  Constant3/1 -> Switch/1
  Switch/1 -> [VBCM_FDCDKCEn_flg]
  VINP_VehicleType_enum/1 -> Equal/1
  VINP_PDKeyAreaPTG_enum/1 -> [VINP_PDKeyAreaPTG_enum]
  [VINP_PDKeyAreaPTG_enum] -> Compare To Constant/1
  [VINP_PDKeyAreaPTG_enum] -> Compare To Constant2/1
  Data Type Conversion7/1 -> Switch5/3
  Compare To Constant2/1 -> Switch5/2
  Switch5/1 -> Switch4/3
  Constant1/1 -> Data Type Conversion1/1
  Data Type Conversion1/1 -> Switch5/1
  task_time_s/1 -> [task_time_s]
  VDKC_KeyAreaSPTGSta_enum/1 -> Switch9/3, Switch7/3, Compare To Constant4/1, Compare To Constant5/1, Detect Change2/1
  Compare To Constant4/1 -> Switch7/2
  Saturation1/1 -> Less Than1/1, Unit Delay2/1
  Constant9/1 -> Less Than1/2
  Add1/1 -> Switch8/3
  [task_time_s] -> Add1/1
  Switch8/1 -> Saturation1/1
  Unit Delay2/1 -> Add1/2
  Data Type Conversion3/1 -> Switch8/1
  Constant10/1 -> Data Type Conversion3/1
  AND1/1 -> Switch8/2
  Compare To Constant5/1 -> AND1/2
  Detect Change2/1 -> AND1/1
  Less Than1/1 -> Switch9/2
  Switch9/1 -> Switch7/1
  Unit Delay3/1 -> Switch9/1
  Switch7/1 -> Switch11/3, Unit Delay3/1
  Divide/1 -> Chart/17(KBCM_SPTGDetectWaitT_s)
  Constant/1 -> Divide/1
  [task_time_s] -> Divide/2
  Switch3/1 -> Chart/7(KeyDetectedOut)
  [VBCM_FDCDKCEn_flg] -> Switch3/2
  KeyDetected/2(KeyDetectedOut) -> Switch3/3
  [VBCM_FDCDKCEn_flg] -> Switch6/2
  Constant5/1 -> Switch6/3
  Constant19/1 -> Switch6/1
  Switch6/1 -> [VBCM_USSFilterT_K]
  [VBCM_USSFilterT_K] -> KeyDetected/2(VBCM_USSFilterT_K)
  Switch10/1 -> Chart/13(KBCM_ReDetectT_K)
  [VBCM_FDCDKCEn_flg] -> Switch10/2
  KBCM_ReDetectT_K/1 -> Switch10/3
  Constant7/1 -> Switch10/1
  Switch11/1 -> Compare To Constant1/1
  Constant11/1 -> Data Type Conversion2/1
  Data Type Conversion2/1 -> Switch11/1
  [SPTGZoneReject] -> AND/1
  Constant12/1 -> AND/2
  AND/1 -> Switch11/2
  [VAPM_PASDRMR_cm] -> Switch1/3
  [VAPM_PASDRML_cm] -> Switch2/3
  [VAPM_PASDRML_cm] -> Compare To Constant3/1
  [VAPM_PASDRMR_cm] -> Compare To Constant6/1
  VAPM_PASDRMR_cm/1 -> Subsystem1/1(VAPM_PASDRMR_cm)
  Subsystem1/1(PASDRMR) -> [VAPM_PASDRMR_cm]  "VBCM_PASDRMRF_cm"
  VAPM_PASDRML_cm/1 -> Subsystem3/1(VAPM_PASDRML_cm)
  Subsystem3/1(PASDRML) -> [VAPM_PASDRML_cm]  "VBCM_PASDRMLF_cm"
  Switch1/1 -> KeyDetected/1(VBCM_PASDRMR_cm), Chart/3(PASDRMR)
  Switch2/1 -> Chart/4(PASDRML), KeyDetected/3(VBCM_PASDRML_cm)
  Compare To Constant3/1 -> OR/2
  Compare To Constant6/1 -> OR/1
  OR/1 -> [SPTGZoneReject]
